simulink model "verify_loeb_spindle"  (Simulink 8.1)
settings: Solver=ode2  StartTime=0.0  StopTime=4  FixedStep=T  RelTol=1e-3
InitFcn:
  | [A tau T] = emg_filter();
  | up = generate_min_jerk( 1, 1.1, 2.0, T );
  | down = 2.1 - up;
  | stretch = [repmat([up; down], 2, 1); [up ;down]];
  | l = length(stretch);
  | stretch(1 : ceil(l/3), 2) = 1;
  | stretch(:, 1) = [0:l-1]*T;
  | 
  | mag1 = 48144;
  | mag2 = 45845;
  | trise = 0.02;
  | tfall  = 0.04;
  | [num_syn den_syn] = filter_coef(mag1, mag2, trise, tfall,T)
  | 
  | for i = 1:20
  | %    eval(['SIZE_MU_', num2str(i), '=', num2str('(atan(150) - atan(i^0.8)) * 6;')])
  | 
  |     eval(['SIZE_MU_', num2str(i), '=', num2str('(atan(150) - atan(2^0.8)) * 6;')])
  | end
StopFcn:
  | %recruitment_pattern_plotter(spikes_g1, spikes_g2, total_force, 0.02)
  | 
  | % Increase the var suffix by 1
  | incrementVars('verify_loeb_spindle')
undefined symbols (not defined in the file or in its folder): SIZE_MU_1, SIZE_MU_10, SIZE_MU_2, SIZE_MU_3, SIZE_MU_4, SIZE_MU_5, SIZE_MU_6, SIZE_MU_7, SIZE_MU_8, SIZE_MU_9, T
libraries: simulink x5
settings Model: Creator=minos_niu  LastModifiedBy=C. Minos Niu
settings DebuggingCC: FcnCallInpInsideContextMsg=EnableAllAsWarning
settings ModelReferenceCC: EnableParallelModelReferenceBuilds=on

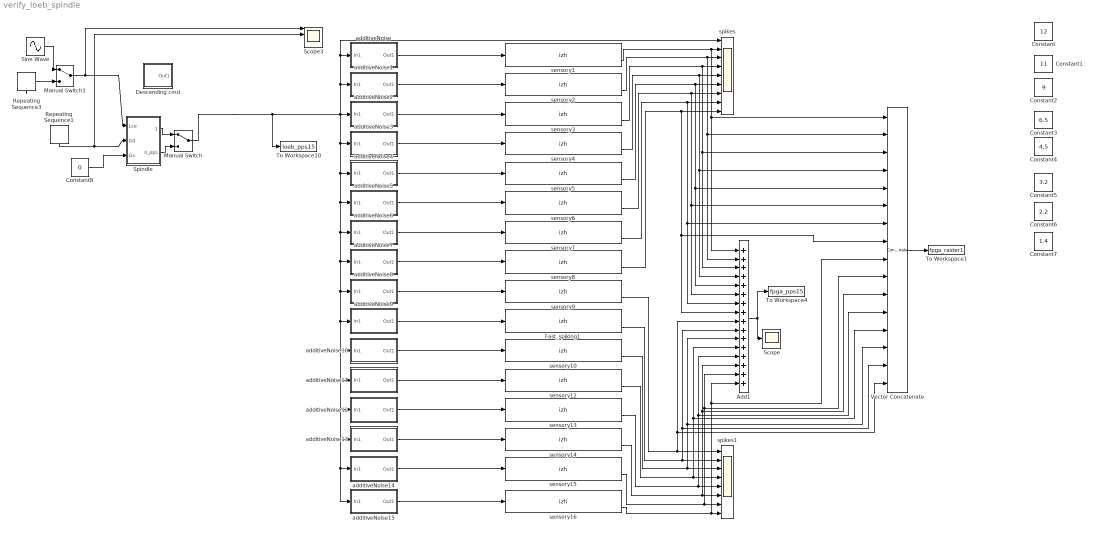
== system verify_loeb_spindle ==
  Add1 : Sum  Inputs=++++++++++++++++
  Constant : Constant  Value=12
  Constant1 : Constant  Value=11
  Constant2 : Constant  Value=9
  Constant3 : Constant  Value=6.5
  Constant4 : Constant  Value=4.5
  Constant5 : Constant  Value=3.2
  Constant6 : Constant  Value=2.2
  Constant7 : Constant  Value=1.4
  Constant8 : Constant  Value=0
  Descending cmd : Subsystem
  Fast_spiking1 : S-Function  FunctionName=izh  Parameters=[0.01 0.2 -65.0 2.0 30.0 SIZE_MU_10] [-70.0 -14.0]  EnableBusSupport=off
      mask Display:
      | port_label('input', 1, 'syn curr');
      | port_label('output', 1, 'action potential');
      | port_label('output', 2, 'spike');
      | disp('Izhi Neuron \n(S-Function)')
  Manual Switch : ManualSwitch
  Manual Switch1 : ManualSwitch
  Repeating Sequence1 : simulink/Sources/Repeating Sequence  rep_seq_t=[0 1.8 2.1 4.0]  rep_seq_y=[1.00 1.0 80.0 80.0]
  Repeating Sequence3 : simulink/Sources/Repeating Sequence  rep_seq_t=[0 1.3 1.5 4.0]  rep_seq_y=[1.00 1.0 1.04 1.04]
  Scope : Scope
      settings: SaveName=ScopeData3
  Scope3 : Scope  NumInputPorts=4
      settings: TimeRange=10  YMin=0~-5~-5~-5  YMax=37.5~5~5~5  SaveName=total_force2  DataFormat=Structure
  Sine Wave : Sin  Amplitude=0.1  Bias=1.1  Frequency=2*pi*2  Phase=-pi/2  SampleTime=T
  Spindle : Subsystem
  To Workspace1 : ToWorkspace  VariableName=fpga_raster1  SampleTime=-1
  To Workspace10 : ToWorkspace  VariableName=loeb_pps15  SampleTime=-1
  To Workspace4 : ToWorkspace  VariableName=fpga_pps15  SampleTime=-1
  Vector Concatenate : Concatenate  NumInputs=16
  additiveNoise : Subsystem  VariantControl=Variant1
  additiveNoise1 : Subsystem  VariantControl=Variant1
  additiveNoise10 : Subsystem  VariantControl=Variant1
  additiveNoise11 : Subsystem  VariantControl=Variant1
  additiveNoise12 : Subsystem  VariantControl=Variant1
  additiveNoise13 : Subsystem  VariantControl=Variant1
  additiveNoise14 : Subsystem  VariantControl=Variant1
  additiveNoise15 : Subsystem  VariantControl=Variant1
  additiveNoise2 : Subsystem  VariantControl=Variant1
  additiveNoise3 : Subsystem  VariantControl=Variant1
  additiveNoise4 : Subsystem  VariantControl=Variant1
  additiveNoise5 : Subsystem  VariantControl=Variant1
  additiveNoise6 : Subsystem  VariantControl=Variant1
  additiveNoise7 : Subsystem  VariantControl=Variant1
  additiveNoise8 : Subsystem  VariantControl=Variant1
  additiveNoise9 : Subsystem  VariantControl=Variant1
  sensory1 : S-Function  FunctionName=izh  Parameters=[0.02 0.2 -65.0 6.0 30.0 SIZE_MU_1] [-70.0 -14.0]  EnableBusSupport=off
      mask Display:
      | port_label('input', 1, 'syn curr');
      | port_label('output', 1, 'action potential');
      | port_label('output', 2, 'spike');
      | disp('Izhi Neuron \n(S-Function)')
  sensory10 : S-Function  FunctionName=izh  Parameters=[0.02 0.2 -65.0 6.0 30.0 SIZE_MU_1] [-70.0 -14.0]  EnableBusSupport=off
      mask Display:
      | port_label('input', 1, 'syn curr');
      | port_label('output', 1, 'action potential');
      | port_label('output', 2, 'spike');
      | disp('Izhi Neuron \n(S-Function)')
  sensory12 : S-Function  FunctionName=izh  Parameters=[0.02 0.2 -65.0 6.0 30.0 SIZE_MU_2] [-70.0 -14.0]  EnableBusSupport=off
      mask Display:
      | port_label('input', 1, 'syn curr');
      | port_label('output', 1, 'action potential');
      | port_label('output', 2, 'spike');
      | disp('Izhi Neuron \n(S-Function)')
  sensory13 : S-Function  FunctionName=izh  Parameters=[0.02 0.2 -65.0 6.0 30.0 SIZE_MU_3] [-70.0 -14.0]  EnableBusSupport=off
      mask Display:
      | port_label('input', 1, 'syn curr');
      | port_label('output', 1, 'action potential');
      | port_label('output', 2, 'spike');
      | disp('Izhi Neuron \n(S-Function)')
  sensory14 : S-Function  FunctionName=izh  Parameters=[0.02 0.2 -65.0 6.0 30.0 SIZE_MU_4] [-70.0 -14.0]  EnableBusSupport=off
      mask Display:
      | port_label('input', 1, 'syn curr');
      | port_label('output', 1, 'action potential');
      | port_label('output', 2, 'spike');
      | disp('Izhi Neuron \n(S-Function)')
  sensory15 : S-Function  FunctionName=izh  Parameters=[0.02 0.2 -65.0 6.0 30.0 SIZE_MU_5] [-70.0 -14.0]  EnableBusSupport=off
      mask Display:
      | port_label('input', 1, 'syn curr');
      | port_label('output', 1, 'action potential');
      | port_label('output', 2, 'spike');
      | disp('Izhi Neuron \n(S-Function)')
  sensory16 : S-Function  FunctionName=izh  Parameters=[0.02 0.2 -65.0 6.0 30.0 SIZE_MU_6] [-70.0 -14.0]  EnableBusSupport=off
      mask Display:
      | port_label('input', 1, 'syn curr');
      | port_label('output', 1, 'action potential');
      | port_label('output', 2, 'spike');
      | disp('Izhi Neuron \n(S-Function)')
  sensory2 : S-Function  FunctionName=izh  Parameters=[0.02 0.2 -65.0 6.0 30.0 SIZE_MU_2] [-70.0 -14.0]  EnableBusSupport=off
      mask Display:
      | port_label('input', 1, 'syn curr');
      | port_label('output', 1, 'action potential');
      | port_label('output', 2, 'spike');
      | disp('Izhi Neuron \n(S-Function)')
  sensory3 : S-Function  FunctionName=izh  Parameters=[0.02 0.2 -65.0 6.0 30.0 SIZE_MU_3] [-70.0 -14.0]  EnableBusSupport=off
      mask Display:
      | port_label('input', 1, 'syn curr');
      | port_label('output', 1, 'action potential');
      | port_label('output', 2, 'spike');
      | disp('Izhi Neuron \n(S-Function)')
  sensory4 : S-Function  FunctionName=izh  Parameters=[0.02 0.2 -65.0 6.0 30.0 SIZE_MU_4] [-70.0 -14.0]  EnableBusSupport=off
      mask Display:
      | port_label('input', 1, 'syn curr');
      | port_label('output', 1, 'action potential');
      | port_label('output', 2, 'spike');
      | disp('Izhi Neuron \n(S-Function)')
  sensory5 : S-Function  FunctionName=izh  Parameters=[0.02 0.2 -65.0 6.0 30.0 SIZE_MU_5] [-70.0 -14.0]  EnableBusSupport=off
      mask Display:
      | port_label('input', 1, 'syn curr');
      | port_label('output', 1, 'action potential');
      | port_label('output', 2, 'spike');
      | disp('Izhi Neuron \n(S-Function)')
  sensory6 : S-Function  FunctionName=izh  Parameters=[0.02 0.2 -65.0 6.0 30.0 SIZE_MU_6] [-70.0 -14.0]  EnableBusSupport=off
      mask Display:
      | port_label('input', 1, 'syn curr');
      | port_label('output', 1, 'action potential');
      | port_label('output', 2, 'spike');
      | disp('Izhi Neuron \n(S-Function)')
  sensory7 : S-Function  FunctionName=izh  Parameters=[0.02 0.2 -65.0 6.0 30.0 SIZE_MU_7] [-70.0 -14.0]  EnableBusSupport=off
      mask Display:
      | port_label('input', 1, 'syn curr');
      | port_label('output', 1, 'action potential');
      | port_label('output', 2, 'spike');
      | disp('Izhi Neuron \n(S-Function)')
  sensory8 : S-Function  FunctionName=izh  Parameters=[0.02 0.2 -65.0 6.0 30.0 SIZE_MU_8] [-70.0 -14.0]  EnableBusSupport=off
      mask Display:
      | port_label('input', 1, 'syn curr');
      | port_label('output', 1, 'action potential');
      | port_label('output', 2, 'spike');
      | disp('Izhi Neuron \n(S-Function)')
  sensory9 : S-Function  FunctionName=izh  Parameters=[0.02 0.2 -65.0 6.0 30.0 SIZE_MU_9] [-70.0 -14.0]  EnableBusSupport=off
      mask Display:
      | port_label('input', 1, 'syn curr');
      | port_label('output', 1, 'action potential');
      | port_label('output', 2, 'spike');
      | disp('Izhi Neuron \n(S-Function)')
  spikes : Scope  NumInputPorts=9
      settings: TickLabels=on  TimeRange=5  YMin=-1000~-5~-5~-5~-5~-5~-5~-5~-5  YMax=5000~5~5~5~5~5~5~5~5  SaveName=spikes_g1  DataFormat=Structure
  spikes1 : Scope  NumInputPorts=8
      settings: TickLabels=on  TimeRange=5  YMin=-1000~-5~-5~-5~-5~-5~-5~-5  YMax=5000~5~5~5~5~5~5~5  SaveName=spikes_g  DataFormat=Structure
  wires:
  sensory1/2 -> Add1/1, Vector Concatenate/1, spikes/2
  sensory2/2 -> Add1/2, Vector Concatenate/2, spikes/3
  sensory3/2 -> Add1/3, Vector Concatenate/3, spikes/4
  sensory4/2 -> Add1/4, Vector Concatenate/4, spikes/5
  sensory5/2 -> Add1/5, Vector Concatenate/5, spikes/6
  sensory6/2 -> Add1/6, Vector Concatenate/6, spikes/7
  sensory7/2 -> Add1/7, Vector Concatenate/7, spikes/8
  additiveNoise/1(Out1) -> sensory1/1
  additiveNoise1/1(Out1) -> sensory2/1
  additiveNoise2/1(Out1) -> sensory3/1
  additiveNoise3/1(Out1) -> sensory4/1
  additiveNoise4/1(Out1) -> sensory5/1
  additiveNoise5/1(Out1) -> sensory6/1
  additiveNoise6/1(Out1) -> sensory7/1
  additiveNoise7/1(Out1) -> sensory8/1
  additiveNoise8/1(Out1) -> sensory9/1
  Constant8/1 -> Spindle/3(Gs)
  Spindle/1(Ia_pps) -> Manual Switch/1
  Spindle/2(II_pps) -> Manual Switch/2
  Manual Switch/1 -> To Workspace10/1, additiveNoise2/1(In1), additiveNoise1/1(In1), spikes/1, additiveNoise/1(In1), additiveNoise3/1(In1), additiveNoise4/1(In1), additiveNoise6/1(In1), additiveNoise7/1(In1), additiveNoise8/1(In1), additiveNoise9/1(In1), additiveNoise15/1(In1), additiveNoise14/1(In1), additiveNoise13/1(In1), additiveNoise12/1(In1), additiveNoise11/1(In1), additiveNoise10/1(In1), additiveNoise5/1(In1)
  Manual Switch1/1 -> Spindle/1(Lce), Scope3/1
  Sine Wave/1 -> Manual Switch1/1
  Repeating Sequence3/1 -> Manual Switch1/2
  Repeating Sequence1/1 -> Spindle/2(Gd), Scope3/2
  additiveNoise9/1(Out1) -> Fast_spiking1/1
  Add1/1 -> To Workspace4/1, Scope/1
  additiveNoise10/1(Out1) -> sensory10/1
  additiveNoise11/1(Out1) -> sensory12/1
  additiveNoise12/1(Out1) -> sensory13/1
  additiveNoise13/1(Out1) -> sensory14/1
  additiveNoise14/1(Out1) -> sensory15/1
  additiveNoise15/1(Out1) -> sensory16/1
  sensory8/2 -> Add1/8, Vector Concatenate/8, spikes/9
  Fast_spiking1/2 -> spikes1/2, Vector Concatenate/15, Add1/10
  sensory10/2 -> spikes1/3, Vector Concatenate/14, Add1/11
  sensory12/2 -> spikes1/4, Vector Concatenate/13, Add1/12
  sensory13/2 -> Vector Concatenate/12, Add1/13, spikes1/5
  sensory15/2 -> Vector Concatenate/10, Add1/15, spikes1/7
  sensory16/2 -> Vector Concatenate/9, Add1/16, spikes1/8
  Vector Concatenate/1 -> To Workspace1/1
  sensory9/2 -> spikes1/1, Add1/9, Vector Concatenate/16
  sensory14/2 -> Vector Concatenate/11, Add1/14, spikes1/6

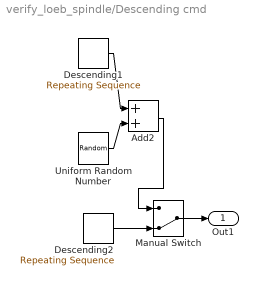
== system verify_loeb_spindle/Descending cmd ==
  Add2 : Sum
  Descending1 : simulink/Sources/Repeating Sequence  rep_seq_t=[0 1.1 3.1 6.8 9.5 10 ]  rep_seq_y=[0 0 20 20 0 0]*1
  Descending2 : simulink/Sources/Repeating Sequence  rep_seq_t=[0 0.5 1]  rep_seq_y=[0 200 200]*0
  Manual Switch : ManualSwitch  CurrentSetting=0
  Uniform Random Number : UniformRandomNumber  Minimum=-6  Maximum=0  SampleTime=T
  Out1 : Outport
  wires:
  Manual Switch/1 -> Out1/1
  Add2/1 -> Manual Switch/1
  Uniform Random Number/1 -> Add2/2
  Descending2/1 -> Manual Switch/2
  Descending1/1 -> Add2/1

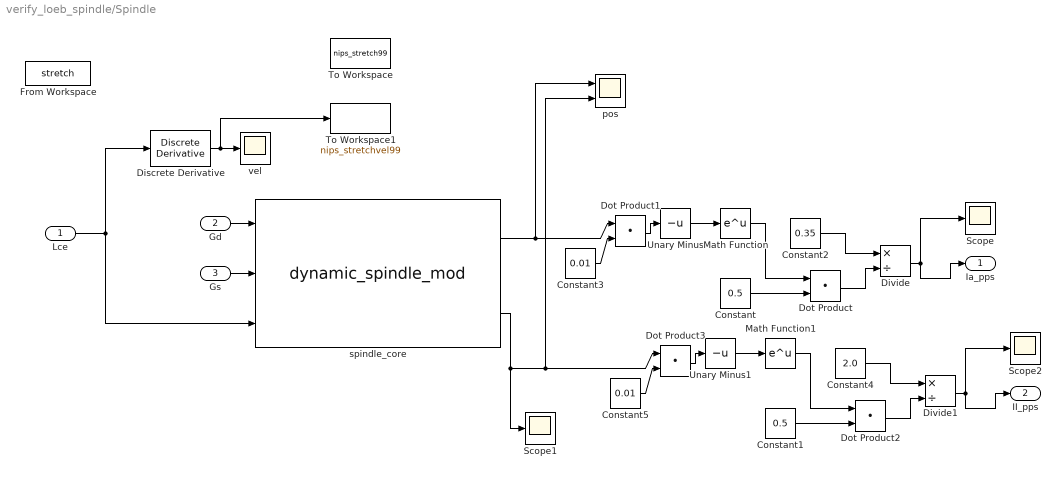
== system verify_loeb_spindle/Spindle ==
  Lce : Inport
  Gd : Inport  Port=2
  Gs : Inport  Port=3
  Constant : Constant  Value=0.5
  Constant1 : Constant  Value=0.5
  Constant2 : Constant  Value=0.35
  Constant3 : Constant  Value=0.01
  Constant4 : Constant  Value=2.0
  Constant5 : Constant  Value=0.01
  Discrete Derivative : simulink/Discrete/Discrete Derivative  gainval=1.0  ICPrevScaledInput=0  InputProcessing=Inherited  OutMin=[]  OutMax=[]  OutDataType=fixdt(1, 16)  OutScaling=2^-10  DoSatur=off
  Divide : Product  Inputs=*/
  Divide1 : Product  Inputs=*/
  Dot Product{,1..3} (4 alike) : DotProduct  InputSameDT=on  OutDataTypeStr=Inherit: Inherit via internal rule
  From Workspace : FromWorkspace  VariableName=stretch  SampleTime=T
  Math Function : Math  SaturateOnIntegerOverflow=on
  Math Function1 : Math  SaturateOnIntegerOverflow=on
  Scope : Scope
      settings: YMin=0  YMax=225
  Scope1 : Scope
      settings: TimeRange=1  SaveName=ScopeData4
  Scope2 : Scope
      settings: YMin=0  YMax=225  SaveName=ScopeData2
  To Workspace : ToWorkspace  VariableName=nips_stretch99  SampleTime=-1  SaveFormat=Structure With Time
  To Workspace1 : ToWorkspace  VariableName=nips_stretchvel99  SampleTime=-1  SaveFormat=Structure With Time
  Unary Minus : UnaryMinus
  Unary Minus1 : UnaryMinus
  pos : Scope  NumInputPorts=2
      settings: YMin=-5~-5  YMax=5~5  SaveName=ScopeData5
  spindle_core : S-Function  FunctionName=dynamic_spindle_mod  Parameters=[10.4649 10.4649 10.4649] [0.1127 0.1623 0.1623] [0.0605 0.0822 0.0822] [0.2356 -0.046 -0.069] [0 0 0] [0.0289 0.0636 0.0954] [1 0.7 0.7] [1 0.92 0.92] [20000 10000 10000] [20000 7250 7250] [0.3 0.3 0.3] [0.46 0.46 0.46] [0.04 0.04 0.04] [0.76 0.76 0.76] [1 0.04 0.04] [0.192 0.185 0.0001] [0.0002 0.0002 0.0002] [1 0.5 1] [1]  EnableBusSupport=off
      mask Display:
      | port_label('input', 1, 'gamma dynamic');
      | port_label('input', 2, 'gamma static');
      | port_label('input', 3, 'Lce(L0)');
      | port_label('output',1,'Ia');
      | port_label('output',2,'II');
      | disp('Muscle Spindle \n(S-Function)')
  vel : Scope
      settings: SaveName=ScopeData6
  Ia_pps : Outport
  II_pps : Outport  Port=2
  wires:
  Discrete Derivative/1 -> vel/1, To Workspace1/1
  spindle_core/1 -> Dot Product1/1, pos/1
  spindle_core/2 -> Scope1/1, Dot Product3/1, pos/2
  Math Function/1 -> Dot Product/1
  Constant/1 -> Dot Product/2
  Unary Minus/1 -> Math Function/1
  Constant2/1 -> Divide/1
  Dot Product/1 -> Divide/2
  Divide/1 -> Ia_pps/1, Scope/1
  Constant3/1 -> Dot Product1/2
  Dot Product1/1 -> Unary Minus/1
  Lce/1 -> Discrete Derivative/1, spindle_core/3
  Gd/1 -> spindle_core/1
  Gs/1 -> spindle_core/2
  Math Function1/1 -> Dot Product2/1
  Constant1/1 -> Dot Product2/2
  Unary Minus1/1 -> Math Function1/1
  Constant4/1 -> Divide1/1
  Dot Product2/1 -> Divide1/2
  Divide1/1 -> II_pps/1, Scope2/1
  Constant5/1 -> Dot Product3/2
  Dot Product3/1 -> Unary Minus1/1

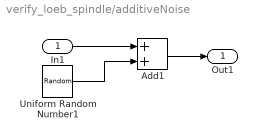
== system verify_loeb_spindle/additiveNoise ==
  In1 : Inport
  Add1 : Sum
  Uniform Random Number1 : UniformRandomNumber  Seed=floor(rand()*100)  SampleTime=T
  Out1 : Outport
  wires:
  Uniform Random Number1/1 -> Add1/2
  In1/1 -> Add1/1
  Add1/1 -> Out1/1

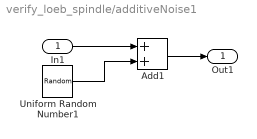
== system verify_loeb_spindle/additiveNoise1 ==
  In1 : Inport
  Add1 : Sum
  Uniform Random Number1 : UniformRandomNumber  Seed=floor(rand()*100)  SampleTime=T
  Out1 : Outport
  wires:
  Add1/1 -> Out1/1
  In1/1 -> Add1/1
  Uniform Random Number1/1 -> Add1/2

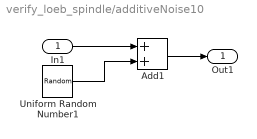
== system verify_loeb_spindle/additiveNoise10 ==
  In1 : Inport
  Add1 : Sum
  Uniform Random Number1 : UniformRandomNumber  Seed=floor(rand()*100)  SampleTime=T
  Out1 : Outport
  wires:
  Uniform Random Number1/1 -> Add1/2
  In1/1 -> Add1/1
  Add1/1 -> Out1/1

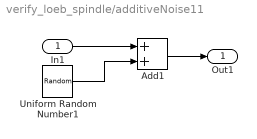
== system verify_loeb_spindle/additiveNoise11 ==
  In1 : Inport
  Add1 : Sum
  Uniform Random Number1 : UniformRandomNumber  Seed=floor(rand()*100)  SampleTime=T
  Out1 : Outport
  wires:
  Add1/1 -> Out1/1
  In1/1 -> Add1/1
  Uniform Random Number1/1 -> Add1/2

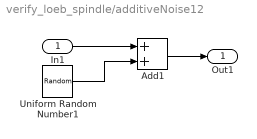
== system verify_loeb_spindle/additiveNoise12 ==
  In1 : Inport
  Add1 : Sum
  Uniform Random Number1 : UniformRandomNumber  Seed=floor(rand()*100)  SampleTime=T
  Out1 : Outport
  wires:
  Uniform Random Number1/1 -> Add1/2
  In1/1 -> Add1/1
  Add1/1 -> Out1/1

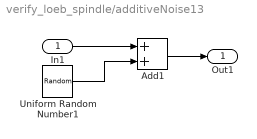
== system verify_loeb_spindle/additiveNoise13 ==
  In1 : Inport
  Add1 : Sum
  Uniform Random Number1 : UniformRandomNumber  Seed=floor(rand()*100)  SampleTime=T
  Out1 : Outport
  wires:
  Add1/1 -> Out1/1
  In1/1 -> Add1/1
  Uniform Random Number1/1 -> Add1/2

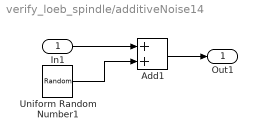
== system verify_loeb_spindle/additiveNoise14 ==
  In1 : Inport
  Add1 : Sum
  Uniform Random Number1 : UniformRandomNumber  Seed=floor(rand()*100)  SampleTime=T
  Out1 : Outport
  wires:
  Add1/1 -> Out1/1
  In1/1 -> Add1/1
  Uniform Random Number1/1 -> Add1/2

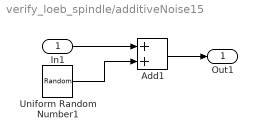
== system verify_loeb_spindle/additiveNoise15 ==
  In1 : Inport
  Add1 : Sum
  Uniform Random Number1 : UniformRandomNumber  Seed=floor(rand()*100)  SampleTime=T
  Out1 : Outport
  wires:
  Uniform Random Number1/1 -> Add1/2
  In1/1 -> Add1/1
  Add1/1 -> Out1/1

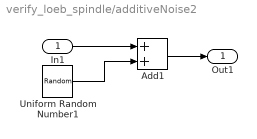
== system verify_loeb_spindle/additiveNoise2 ==
  In1 : Inport
  Add1 : Sum
  Uniform Random Number1 : UniformRandomNumber  Seed=floor(rand()*100)  SampleTime=T
  Out1 : Outport
  wires:
  Add1/1 -> Out1/1
  In1/1 -> Add1/1
  Uniform Random Number1/1 -> Add1/2

== system verify_loeb_spindle/additiveNoise3 ==
  In1 : Inport
  Add1 : Sum
  Uniform Random Number1 : UniformRandomNumber  Seed=floor(rand()*100)  SampleTime=T
  Out1 : Outport
  wires:
  Uniform Random Number1/1 -> Add1/2
  In1/1 -> Add1/1
  Add1/1 -> Out1/1

== system verify_loeb_spindle/additiveNoise4 ==
  In1 : Inport
  Add1 : Sum
  Uniform Random Number1 : UniformRandomNumber  Seed=floor(rand()*100)  SampleTime=T
  Out1 : Outport
  wires:
  Add1/1 -> Out1/1
  In1/1 -> Add1/1
  Uniform Random Number1/1 -> Add1/2

== system verify_loeb_spindle/additiveNoise5 ==
  In1 : Inport
  Add1 : Sum
  Uniform Random Number1 : UniformRandomNumber  Seed=floor(rand()*100)  SampleTime=T
  Out1 : Outport
  wires:
  Uniform Random Number1/1 -> Add1/2
  In1/1 -> Add1/1
  Add1/1 -> Out1/1

== system verify_loeb_spindle/additiveNoise6 ==
  In1 : Inport
  Add1 : Sum
  Uniform Random Number1 : UniformRandomNumber  Seed=floor(rand()*100)  SampleTime=T
  Out1 : Outport
  wires:
  Uniform Random Number1/1 -> Add1/2
  In1/1 -> Add1/1
  Add1/1 -> Out1/1

== system verify_loeb_spindle/additiveNoise7 ==
  In1 : Inport
  Add1 : Sum
  Uniform Random Number1 : UniformRandomNumber  Seed=floor(rand()*100)  SampleTime=T
  Out1 : Outport
  wires:
  Add1/1 -> Out1/1
  In1/1 -> Add1/1
  Uniform Random Number1/1 -> Add1/2

== system verify_loeb_spindle/additiveNoise8 ==
  In1 : Inport
  Add1 : Sum
  Uniform Random Number1 : UniformRandomNumber  Seed=floor(rand()*100)  SampleTime=T
  Out1 : Outport
  wires:
  Add1/1 -> Out1/1
  In1/1 -> Add1/1
  Uniform Random Number1/1 -> Add1/2

== system verify_loeb_spindle/additiveNoise9 ==
  In1 : Inport
  Add1 : Sum
  Uniform Random Number1 : UniformRandomNumber  Seed=floor(rand()*100)  SampleTime=T
  Out1 : Outport
  wires:
  Uniform Random Number1/1 -> Add1/2
  In1/1 -> Add1/1
  Add1/1 -> Out1/1
